simulink library "conversionsLib"  (R2021b)
settings: Solver=VariableStepAuto  StartTime=0.0  StopTime=10.0  RelTol=1e-3
settings Model: Creator=mat  LastModifiedBy=mat

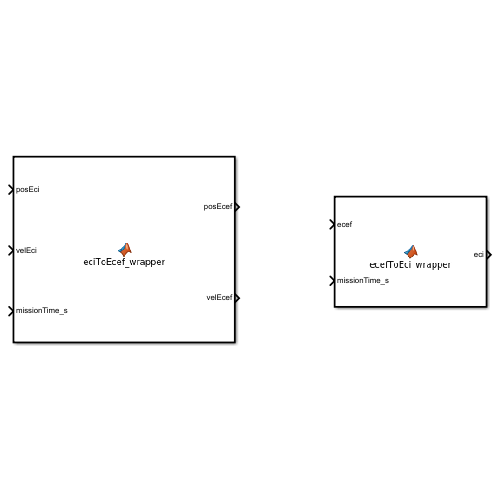
[thumbnail: Simulink's stored preview of the top-level diagram]
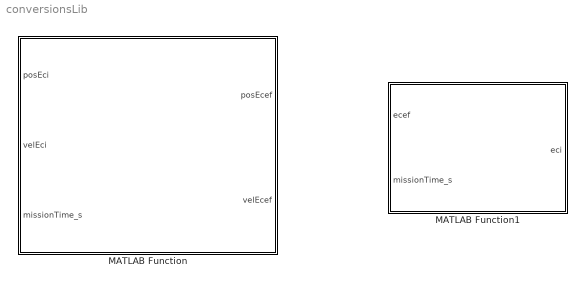
== system conversionsLib ==
  MATLAB Function : MATLAB Function  TreatAsAtomicUnit=on
  MATLAB Function1 : MATLAB Function  TreatAsAtomicUnit=on

== matlab function conversionsLib/MATLAB Function1 ==
  data: ecef input; eci output; missionTime_s input
function eci  = ecefToEci_wrapper(ecef, missionTime_s)

    eci = ecefToEci(ecef, missionTime_s);

end

== matlab function conversionsLib/MATLAB Function ==
  data: posEci input; velEci input; posEcef output; missionTime_s input; velEcef output
function [posEcef, velEcef]  = eciToEcef_wrapper(posEci, velEci ,missionTime_s)

    [posEcef, velEcef] = eciToEcef(posEci, velEci, missionTime_s);

end
